simulink model "fmi_test_GRT_2"  (R2022b)
settings: Solver=FixedStepAuto  StartTime=0.0  StopTime=10.0  RelTol=1e-3
settings Model: Creator=lordx  LastModifiedBy=lordx
settings OptimizationCC: EnableMemcpy=off
settings RTWCC: Description=FMU based on GRT (Functional Mock-up Unit)  SystemTargetFile=grtfmi.tlc  GenerateMakefile=off  TemplateMakefile=none  GenerateReport=on  RetainRTWFile=on
settings CodeAppCC: ForceParamTrailComments=on  StateflowObjectComments=on  MATLABSourceComments=on
settings STFCustomTargetCC: TargetLangStandard=C99 (ISO)  CombineOutputUpdateFcns=on  SystemTargetFile=grtfmi.tlc
settings GRTTargetCC: ParMdlRefBuildCompliant=off  CompOptLevelCompliant=off  ConcurrentExecutionCompliant=off  MatFileLogging=off  CPPClassGenCompliant=off  UseToolchainInfoCompliant=off  RTWCAPISignals=on  RTWCAPIParams=on  RTWCAPIStates=on  RTWCAPIRootIO=on
settings SimscapeCC: SimscapeNormalizeSystem=off

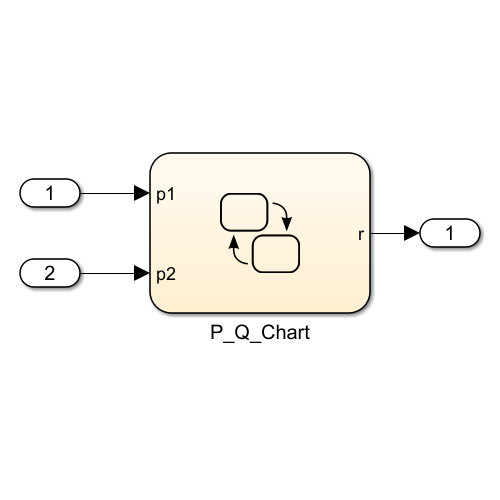
[thumbnail: Simulink's stored preview of the top-level diagram]
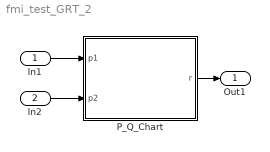
== system fmi_test_GRT_2 ==
  In1 : Inport
  In2 : Inport  Port=2
  P_Q_Chart : Stateflow chart  TreatAsAtomicUnit=on
  Out1 : Outport
  wires:
  P_Q_Chart/1(r) -> Out1/1
  In1/1 -> P_Q_Chart/1(p1)
  In2/1 -> P_Q_Chart/2(p2)

== stateflow chart fmi_test_GRT_2/P_Q_Chart ==
  state init = initialize_fun(p,q,r) [function]
    (default) -> (junction 30) : {
        | q = 0;
        | p = 0;
        | r = 0;
        | }
  state qf = quotient_fun (p1,p2) [function]
    (default) -> (junction 18) : {
        | quotient = p1 / p2;
        | result = quotient;
        | }
  state pf = product_fun(p1,p2) [function]
    (default) -> (junction 23) : {
        | product = p1*p2;
        | result = product;
        | }
  (default) -> (junction 1) : {
      | init = initialize_fun(p,q,r);
      | }
  (junction 1) -> (junction 4) [order 1]
  (junction 1) -> (junction 2) [order 2] : [
      | p1 <= p2
      | ]
      |
      | {
      | r = product_fun(p1,p2);
      | }
  (junction 4) -> (junction 6) : [
      | p1 >= p2
      | ]
      |
      | {
      | r = quotient_fun(p1,p2);
      | }
  (junction 6) -> (junction 2)
  data: p function_input double; init function_output double; q function_input double; r function_input double; p1 function_input double; p2 function_input double; qf function_output double; p1 function_input double; p2 function_input double; pf function_output double; p1 input; p2 input double; quotient local double; product local double; r output double; p local double; q local double; result local double; init local double
